simulink model "week06_robot_model"  (R2026a)
settings: Solver=ode45  StopTime=robot.stopTime  MaxStep=robot.maxStep  RelTol=robot.relativeTolerance  AbsTol=robot.absoluteTolerance
model workspace (MAT data in the model file):
  robot.trackWidth = 0.14
  robot.initialDistance = 0
  robot.initialAngle = 0
  robot.stopTime = 3
  robot.relativeTolerance = 1e-06
  robot.absoluteTolerance = 1e-09
  robot.maxStep = 0.0001
  wheels(1).L = 0.00768482381376
  wheels(1).R = 6.41139804096
  wheels(1).Kt = 0.0102935612741
  wheels(1).Kb = 0.0102935612741
  wheels(1).J = 5.4618603579e-06
  wheels(1).D = 6.52401278375e-07
  wheels(1).gear = 9.68
  wheels(1).wheelRadius = 0.03
  wheels(1).Kp = 2.03180408642
  wheels(1).Ts = 0.001
  wheels(1).voltageLimit = 9
  wheels(1).initialMotorSpeed = 0
  wheels(1).initialCurrent = 0
  wheels(1).initialSensorSpeed = 0
  wheels(1).diagnosticVoltageScale = 0.1
  wheels(2).L = 0.00332761119549
  wheels(2).R = 2.86396181384
  wheels(2).Kt = 0.00798363352314
  wheels(2).Kb = 0.00798363352314
  wheels(2).J = 5.4618603579e-06
  wheels(2).D = 3.3790070145e-06
  wheels(2).gear = 9.68
  wheels(2).wheelRadius = 0.03
  wheels(2).Kp = 0.766619928019
  wheels(2).Ts = 0.001
  wheels(2).voltageLimit = 9
  wheels(2).initialMotorSpeed = 0
  wheels(2).initialCurrent = 0
  wheels(2).initialSensorSpeed = 0
  wheels(2).diagnosticVoltageScale = 0.1
values from neighbouring files (symbols this model uses):
  robot = struct('trackWidth',0.14,'initialDistance',0,'initialAngle',0,      'stopTime',3,'relativeTolerance',1e-6,'absoluteTolerance',1e-9,      'maxStep',min([wheels.Ts])/10)    [robot_model_defaults.m]
  wheels =     [basebot_test_results.mat]    (also in robot_model_defaults.m = tuned.motorParameters; run_basebot_test.m = repmat(struct('L',0,'R',0,'Kt',0,'Kb',0,'J',0,'D',0,      'g)
settings Model: Creator=michaeljohansen  LastModifiedBy=michaeljohansen

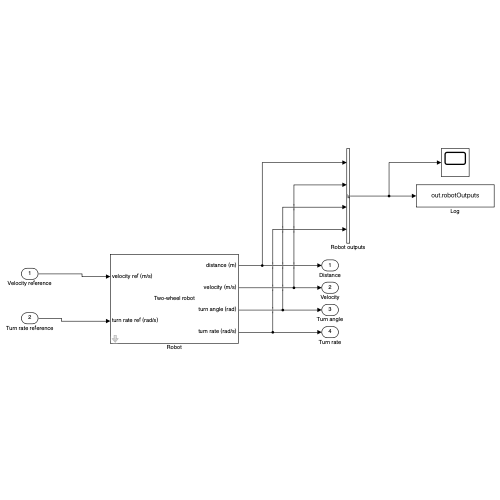
[thumbnail: Simulink's stored preview of the top-level diagram]
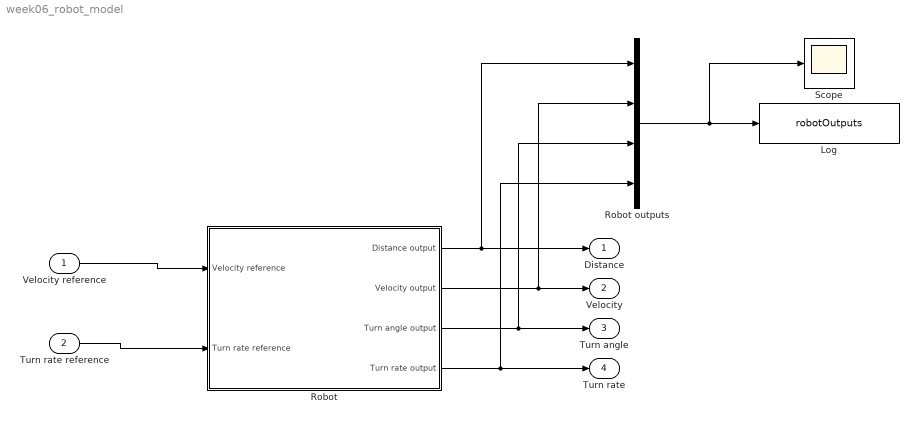
== system week06_robot_model ==
  Velocity reference : Inport
  Turn rate reference : Inport  Port=2
  Log : ToWorkspace  VariableName=robotOutputs  SaveFormat=Timeseries  SampleTime=-1
  Robot : Subsystem  mask{wheelParameters=wheels, robotParameters=robot}
      mask prompts: wheelParameters "Left/right wheel structures"; robotParameters "Robot structure"
      mask Display: disp('Two-wheel robot'); port_label('input',1,'velocity ref (m/s)'); port_label('input',2,'turn rate ref (rad/s)'); port_label('output',1,'distance (m)'); port_label('output',2,'velocity (m/s)'); port_label('output',3,'turn angle (rad)'); port_label('output',4,'turn rate (rad/s)');
  Robot outputs : Mux
  Scope : Scope
  Distance : Outport
  Velocity : Outport  Port=2
  Turn angle : Outport  Port=3
  Turn rate : Outport  Port=4
  wires:
  Robot/1(Distance output) -> Robot outputs/1, Distance/1
  Robot/2(Velocity output) -> Velocity/1, Robot outputs/2
  Robot/3(Turn angle output) -> Turn angle/1, Robot outputs/3
  Robot/4(Turn rate output) -> Turn rate/1, Robot outputs/4
  Velocity reference/1 -> Robot/1(Velocity reference)
  Turn rate reference/1 -> Robot/2(Turn rate reference)
  Robot outputs/1 -> Log/1, Scope/1

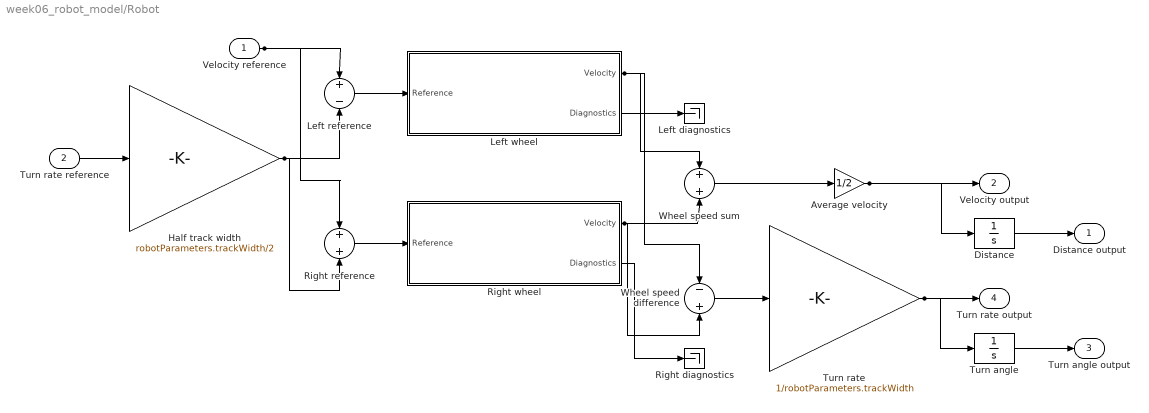
== system week06_robot_model/Robot ==
  Velocity reference : Inport
  Turn rate reference : Inport  Port=2
  Average velocity : Gain  Gain=1/2
  Distance : Integrator  InitialCondition=robotParameters.initialDistance
  Half track width : Gain  Gain=robotParameters.trackWidth/2
  Left diagnostics : Terminator
  Left reference : Sum  Inputs=+-
  Left wheel : Subsystem  mask{L=wheelParameters(1).L, R=wheelParameters(1).R, Kt=wheelParameters(1).Kt, Kb=wheelParameters(1).Kb, J=wheelParameters(1).J, D=wheelParameters(1).D, gear=wheelParameters(1).gear, wheelRadius=wheelParameters(1).wheelRadius, Kp=wheelParameters(1).Kp, Ts=wheelParameters(1).Ts, voltageLimit=wheelParameters(1).voltageLimit, initialMotorSpeed=wheelParameters(1).initialMotorSpeed, initialCurrent=wheelParameters(1).initialCurrent, initialSensorSpeed=wheelParameters(1).initialSensorSpeed, diagnosticVoltageScale=wheelParameters(1).diagnosticVoltageScale}
      mask Display: disp('P-controlled wheel'); port_label('input',1,'reference (m/s)'); port_label('output',1,'velocity (m/s)'); port_label('output',2,'diagnostics');
  Right diagnostics : Terminator
  Right reference : Sum
  Right wheel : Subsystem  mask{L=wheelParameters(2).L, R=wheelParameters(2).R, Kt=wheelParameters(2).Kt, Kb=wheelParameters(2).Kb, J=wheelParameters(2).J, D=wheelParameters(2).D, gear=wheelParameters(2).gear, wheelRadius=wheelParameters(2).wheelRadius, Kp=wheelParameters(2).Kp, Ts=wheelParameters(2).Ts, voltageLimit=wheelParameters(2).voltageLimit, initialMotorSpeed=wheelParameters(2).initialMotorSpeed, initialCurrent=wheelParameters(2).initialCurrent, initialSensorSpeed=wheelParameters(2).initialSensorSpeed, diagnosticVoltageScale=wheelParameters(2).diagnosticVoltageScale}
      mask Display: disp('P-controlled wheel'); port_label('input',1,'reference (m/s)'); port_label('output',1,'velocity (m/s)'); port_label('output',2,'diagnostics');
  Turn angle : Integrator  InitialCondition=robotParameters.initialAngle
  Turn rate : Gain  Gain=1/robotParameters.trackWidth
  Wheel speed difference : Sum  Inputs=-+
  Wheel speed sum : Sum
  Distance output : Outport
  Velocity output : Outport  Port=2
  Turn angle output : Outport  Port=3
  Turn rate output : Outport  Port=4
  wires:
  Turn angle/1 -> Turn angle output/1
  Distance/1 -> Distance output/1
  Average velocity/1 -> Velocity output/1, Distance/1
  Left reference/1 -> Left wheel/1(Reference)
  Wheel speed difference/1 -> Turn rate/1
  Half track width/1 -> Right reference/2, Left reference/2
  Wheel speed sum/1 -> Average velocity/1
  Right wheel/2(Diagnostics) -> Right diagnostics/1
  Right wheel/1(Velocity) -> Wheel speed difference/2, Wheel speed sum/2
  Left wheel/2(Diagnostics) -> Left diagnostics/1
  Left wheel/1(Velocity) -> Wheel speed difference/1, Wheel speed sum/1
  Turn rate/1 -> Turn rate output/1, Turn angle/1
  Velocity reference/1 -> Left reference/1, Right reference/1
  Right reference/1 -> Right wheel/1(Reference)
  Turn rate reference/1 -> Half track width/1

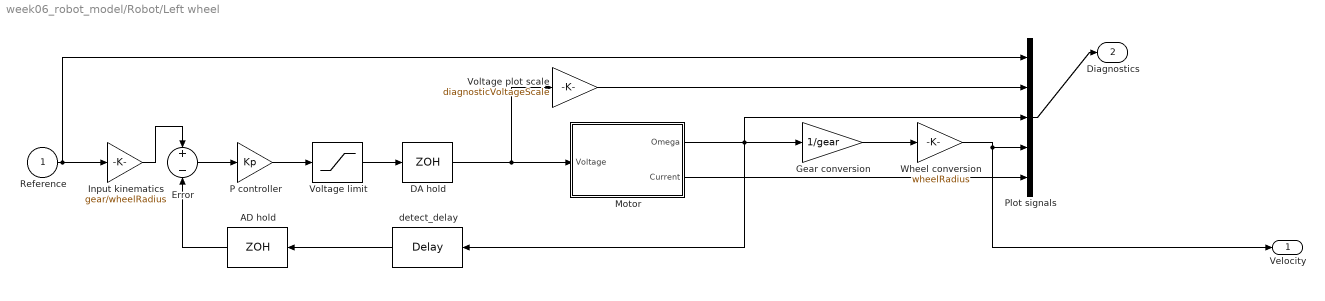
== system week06_robot_model/Robot/Left wheel ==
  Reference : Inport
  AD hold : ZeroOrderHold  SampleTime=Ts
  DA hold : ZeroOrderHold  SampleTime=Ts
  Error : Sum  Inputs=+-
  Gear conversion : Gain  Gain=1/gear
  Input kinematics : Gain  Gain=gear/wheelRadius
  Motor : Subsystem
  P controller : Gain  Gain=Kp
  Plot signals : Mux  Inputs=5
  Voltage limit : Saturate  UpperLimit=voltageLimit  LowerLimit=-voltageLimit
  Voltage plot scale : Gain  Gain=diagnosticVoltageScale
  Wheel conversion : Gain  Gain=wheelRadius
  detect_delay : TransportDelay  DelayTime=Ts  InitialOutput=initialSensorSpeed
  Velocity : Outport
  Diagnostics : Outport  Port=2
  wires:
  Plot signals/1 -> Diagnostics/1
  Reference/1 -> Plot signals/1, Input kinematics/1
  Motor/2(Current) -> Plot signals/5
  Wheel conversion/1 -> Velocity/1, Plot signals/4
  Motor/1(Omega) -> detect_delay/1, Gear conversion/1, Plot signals/3
  Voltage limit/1 -> DA hold/1
  detect_delay/1 -> AD hold/1
  Input kinematics/1 -> Error/1
  Gear conversion/1 -> Wheel conversion/1
  AD hold/1 -> Error/2
  DA hold/1 -> Motor/1(Voltage), Voltage plot scale/1
  Voltage plot scale/1 -> Plot signals/2
  Error/1 -> P controller/1
  P controller/1 -> Voltage limit/1

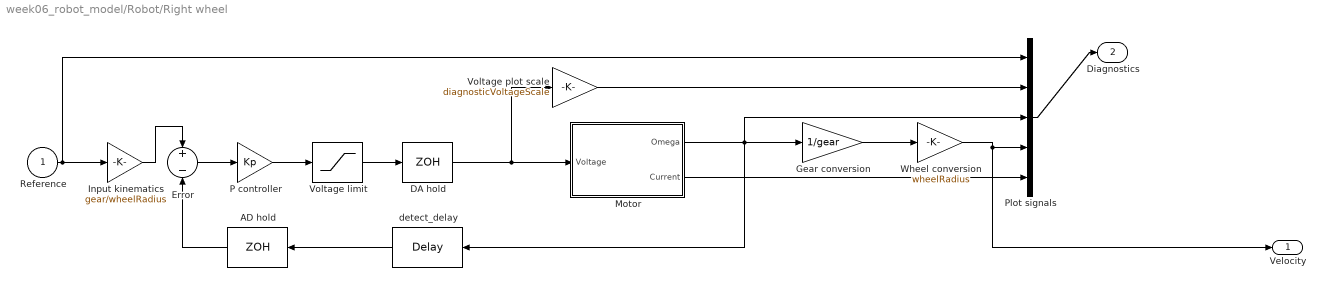
== system week06_robot_model/Robot/Right wheel ==
  Reference : Inport
  AD hold : ZeroOrderHold  SampleTime=Ts
  DA hold : ZeroOrderHold  SampleTime=Ts
  Error : Sum  Inputs=+-
  Gear conversion : Gain  Gain=1/gear
  Input kinematics : Gain  Gain=gear/wheelRadius
  Motor : Subsystem
  P controller : Gain  Gain=Kp
  Plot signals : Mux  Inputs=5
  Voltage limit : Saturate  UpperLimit=voltageLimit  LowerLimit=-voltageLimit
  Voltage plot scale : Gain  Gain=diagnosticVoltageScale
  Wheel conversion : Gain  Gain=wheelRadius
  detect_delay : TransportDelay  DelayTime=Ts  InitialOutput=initialSensorSpeed
  Velocity : Outport
  Diagnostics : Outport  Port=2
  wires:
  Plot signals/1 -> Diagnostics/1
  Reference/1 -> Plot signals/1, Input kinematics/1
  Motor/2(Current) -> Plot signals/5
  Wheel conversion/1 -> Velocity/1, Plot signals/4
  Motor/1(Omega) -> detect_delay/1, Gear conversion/1, Plot signals/3
  Voltage limit/1 -> DA hold/1
  detect_delay/1 -> AD hold/1
  Input kinematics/1 -> Error/1
  Gear conversion/1 -> Wheel conversion/1
  AD hold/1 -> Error/2
  DA hold/1 -> Motor/1(Voltage), Voltage plot scale/1
  Voltage plot scale/1 -> Plot signals/2
  Error/1 -> P controller/1
  P controller/1 -> Voltage limit/1

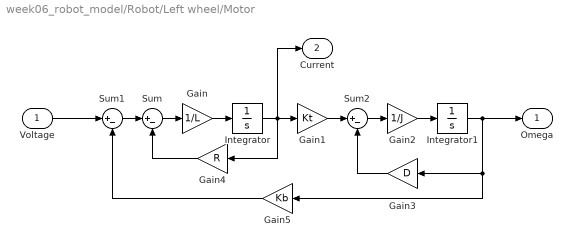
== system week06_robot_model/Robot/Left wheel/Motor ==
  Voltage : Inport
  Gain : Gain  Gain=1/L
  Gain1 : Gain  Gain=Kt
  Gain2 : Gain  Gain=1/J
  Gain3 : Gain  Gain=D
  Gain4 : Gain  Gain=R
  Gain5 : Gain  Gain=Kb
  Integrator : Integrator  InitialCondition=initialCurrent
  Integrator1 : Integrator  InitialCondition=initialMotorSpeed
  Sum : Sum  Inputs=|+-
  Sum1 : Sum  Inputs=|+-
  Sum2 : Sum  Inputs=|+-
  Omega : Outport
  Current : Outport  Port=2
  wires:
  Voltage/1 -> Sum1/1
  Sum1/1 -> Sum/1
  Sum/1 -> Gain/1
  Gain/1 -> Integrator/1
  Integrator/1 -> Gain1/1, Gain4/1, Current/1
  Gain4/1 -> Sum/2
  Gain1/1 -> Sum2/1
  Sum2/1 -> Gain2/1
  Gain2/1 -> Integrator1/1
  Integrator1/1 -> Gain3/1, Gain5/1, Omega/1
  Gain3/1 -> Sum2/2
  Gain5/1 -> Sum1/2

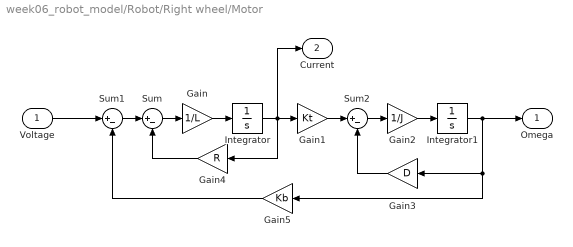
== system week06_robot_model/Robot/Right wheel/Motor ==
  Voltage : Inport
  Gain : Gain  Gain=1/L
  Gain1 : Gain  Gain=Kt
  Gain2 : Gain  Gain=1/J
  Gain3 : Gain  Gain=D
  Gain4 : Gain  Gain=R
  Gain5 : Gain  Gain=Kb
  Integrator : Integrator  InitialCondition=initialCurrent
  Integrator1 : Integrator  InitialCondition=initialMotorSpeed
  Sum : Sum  Inputs=|+-
  Sum1 : Sum  Inputs=|+-
  Sum2 : Sum  Inputs=|+-
  Omega : Outport
  Current : Outport  Port=2
  wires:
  Voltage/1 -> Sum1/1
  Sum1/1 -> Sum/1
  Sum/1 -> Gain/1
  Gain/1 -> Integrator/1
  Integrator/1 -> Gain1/1, Gain4/1, Current/1
  Gain4/1 -> Sum/2
  Gain1/1 -> Sum2/1
  Sum2/1 -> Gain2/1
  Gain2/1 -> Integrator1/1
  Integrator1/1 -> Gain3/1, Gain5/1, Omega/1
  Gain3/1 -> Sum2/2
  Gain5/1 -> Sum1/2
